simulink model "12_pulse_monopolar"  (R2021a)
settings: Solver=VariableStepAuto  StartTime=0.0  StopTime=2  MaxStep=1e-6  RelTol=1e-3
values from neighbouring files (symbols this model uses):
  alpha_i = 180 - gamma_min - mu    (= 160)    [link_params.m]
  alpha_r = 5    [link_params.m]
  V_AC_A = Vl_rms_A*ratio    (= 220000)    [link_params.m]
  V_AC_B = Vl_rms_B*ratio    (= 200000)    [link_params.m]
  Vl_rms_A = 22e3    (= 22000)    [link_params.m]
  Vl_rms_B = 20e3    (= 20000)    [link_params.m]
undefined symbols (not defined in the file or in its folder): D1, Delta, lagging, pulse
libraries: spsUniversalBridgeLib x4, spsSeriesRLCBranchLib x3, spsGroundLib x2, spsPLL3phLib x2, spsThreePhaseVIMeasurementLib x2, spsPulseGeneratorThyristor6PulseLib x2, spsTHDLib x2, spsThreePhaseTransformerThreeWindingsLib x2, spsThreePhaseSourceLib x2, spsVoltageMeasurementLib x2, spsCurrentMeasurementLib x1, spsMultimeterLib x1
settings Model: SimulationMode=accelerator  Creator=HossamAladdin  LastModifiedBy=HossamAladdin
settings DataIOCC: ReturnWorkspaceOutputs=off

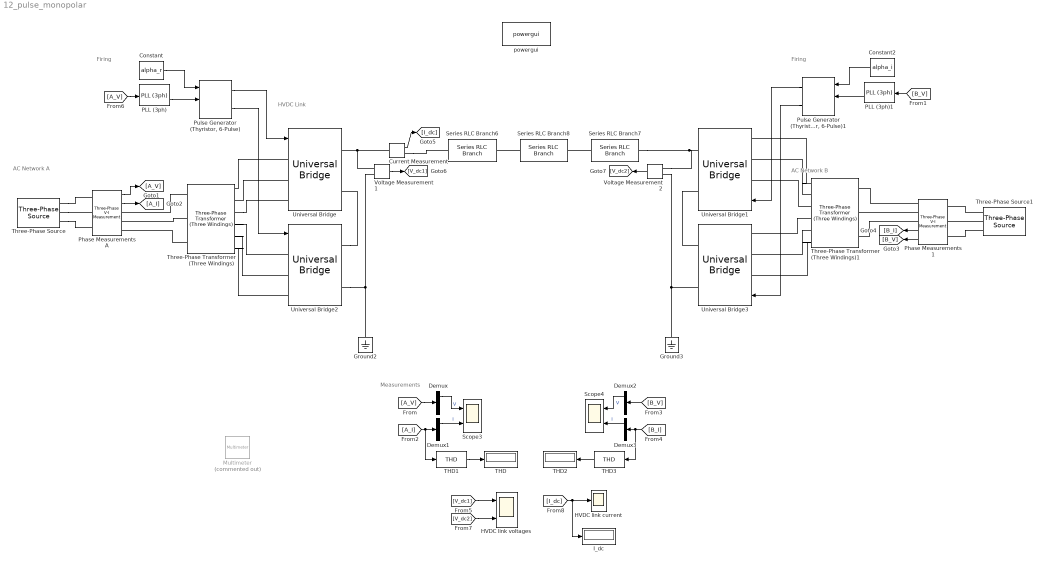
== system 12_pulse_monopolar ==
  note: Measurements
  note: HVDC Link
  note: AC Network A
  note: Firing
  note: AC Network B
  note: Firing
  Constant : Constant  Value=alpha_r
  Constant2 : Constant  Value=alpha_i
  Current Measurement : spsCurrentMeasurementLib/Current Measurement  PhasorSimulation=off  OutputType=Complex  PSBequivalent=0
  Demux{,1..3} (4 alike) : Demux  Outputs=3
  Ground2 : spsGroundLib/Ground  LConnTagsString=a
  Ground3 : spsGroundLib/Ground  LConnTagsString=a
  HVDC link current : Scope
  HVDC link voltages : Scope  NumInputPorts=2
  I_dc : Display
  Multimeter : spsMultimeterLib/Multimeter  Commented=on  PhasorSimulation=off  OutputType=Complex  sel=[1 7 11]  L=16  Gain=[1 1 1]  yselected={'Usw1: Universal Bridge1','Uab: Universal Bridge1','Isw1: Universal Bridge1'};  PSBOutputType=1  PSBequivalent=0  AxesSetting=[0,0.1,-100,100]  Display=1  SavedBlockNames=-11
  PLL (3ph) : spsPLL3phLib/PLL (3ph)  Fmin=50  Par_Init=[0, 50]  ParK=[180, 3200, 1]  TcD=1e-4  MaxRateChangeFreq=12  FilterCutOffFreq=25  Ts=0  AGC=on
  PLL (3ph)1 : spsPLL3phLib/PLL (3ph)  Fmin=60  Par_Init=[0, 60]  ParK=[180, 3200, 1]  TcD=1e-4  MaxRateChangeFreq=12  FilterCutOffFreq=25  Ts=0  AGC=on
  Phase Measurements A : spsThreePhaseVIMeasurementLib/Three-Phase V-I Measurement  VoltageMeasurement=phase-to-ground  SetLabelV=off  LabelV=Vabc  Vpu=off  VpuLL=off  CurrentMeasurement=yes  SetLabelI=off  LabelI=Iabc  Ipu=off  Pbase=100e6  Vbase=500e3  OutputType=Complex  PhasorSimulation=off  PSBequivalent=0
  Phase Measurements1 : spsThreePhaseVIMeasurementLib/Three-Phase V-I Measurement  VoltageMeasurement=phase-to-ground  SetLabelV=off  LabelV=Vabc  Vpu=off  VpuLL=off  CurrentMeasurement=yes  SetLabelI=off  LabelI=Iabc  Ipu=off  Pbase=100e6  Vbase=500e3  OutputType=Complex  PhasorSimulation=off  PSBequivalent=0
  "Pulse Generator (Thyristor, 6-Pulse)" : spsPulseGeneratorThyristor6PulseLib/Pulse Generator (Thyristor, 6-Pulse)  GenType=12-pulse  Delta=D1 (lagging)  pwidth=60  Double_Pulse=off  Ts=0
      settings: SourceProductBaseCode=PS
  "Pulse Generator (Thyristor, 6-Pulse)1" : spsPulseGeneratorThyristor6PulseLib/Pulse Generator (Thyristor, 6-Pulse)  GenType=12-pulse  Delta=D1 (lagging)  pwidth=60  Double_Pulse=off  Ts=0
      settings: SourceProductBaseCode=PS
  Scope3 : Scope  NumInputPorts=2
  Scope4 : Scope  NumInputPorts=2
  Series RLC Branch6 : spsSeriesRLCBranchLib/Series RLC Branch  LConnTagsString=__new0  RConnTagsString=__new0  BranchType=L  Resistance=1  Inductance=1.5  SetiL0=off  InitialCurrent=0  Capacitance=1e-6  Setx0=off  InitialVoltage=0  Measurements=None
  Series RLC Branch7 : spsSeriesRLCBranchLib/Series RLC Branch  LConnTagsString=__new0  RConnTagsString=__new0  BranchType=L  Resistance=1  Inductance=1.5  SetiL0=off  InitialCurrent=0  Capacitance=1e-6  Setx0=off  InitialVoltage=0  Measurements=None
  Series RLC Branch8 : spsSeriesRLCBranchLib/Series RLC Branch  LConnTagsString=__new0  RConnTagsString=__new0  BranchType=R  Resistance=10  Inductance=10e-3  SetiL0=off  InitialCurrent=0  Capacitance=1e-6  Setx0=off  InitialVoltage=0  Measurements=None
  THD : Display
  THD1 : spsTHDLib/THD  Freq=50  Ts=0
      settings: SourceProductBaseCode=PS
  THD2 : Display
  THD3 : spsTHDLib/THD  Freq=50  Ts=0
      settings: SourceProductBaseCode=PS
  Three-Phase Transformer (Three Windings) : spsThreePhaseTransformerThreeWindingsLib/Three-Phase Transformer (Three Windings)  Winding1Connection=Y  Winding2Connection=Y  Winding3Connection=Delta (D1)  CoreType=Three single-phase transformers  SetSaturation=off  Hysteresis=off  DataFile='hysteresis'  SetInitialFlux=off  Measurements=None  UNITS=SI  NominalPower=[ 1000e6 , 50 ]  Winding1=[Vl_rms_A 0 0]  Winding2=[V_AC_A/2 0 0]  Winding3=[V_AC_A/2 0.001 0]  Rm=inf  Lm=inf  L0=0.5  Saturation=[0 0;89.072 68.613;37113 86.91]  InitialFluxes=[-57.1777654238029 28.5888827119015 28.5888827119015]  BreakLoop=off  DiscreteSolver=Trapezoidal iterative  DataType=on  TransfoNumber=1
      settings: SourceProductBaseCode=PS
  Three-Phase Transformer (Three Windings)1 : spsThreePhaseTransformerThreeWindingsLib/Three-Phase Transformer (Three Windings)  Winding1Connection=Y  Winding2Connection=Delta (D1)  Winding3Connection=Y  CoreType=Three single-phase transformers  SetSaturation=off  Hysteresis=off  DataFile='hysteresis'  SetInitialFlux=off  Measurements=None  UNITS=SI  NominalPower=[ 1000e6 , 60 ]  Winding1=[Vl_rms_B 0 0]  Winding2=[V_AC_B/2 0.001 0]  Winding3=[V_AC_B/2 0 0]  Rm=inf  Lm=inf  L0=0.5  Saturation=[0 0;97.98 51.98;40825 65.841]  InitialFluxes=[0 64.9747334361397 64.9747334361397]  BreakLoop=off  DiscreteSolver=Trapezoidal iterative  DataType=on  TransfoNumber=1
      settings: SourceProductBaseCode=PS
  Three-Phase Source : spsThreePhaseSourceLib/Three-Phase Source  InternalConnection=Yg  VoltagePhases=off  Voltage=Vl_rms_A  PhaseAngle=0  Voltage_phases=[25e3 25e3 25e3]/sqrt(3)  PhaseAngles_phases=[0 -120 +120]  Frequency=50  NonIdealSource=off  SpecifyImpedance=off  Resistance=0.8929  Inductance=16.58e-3  ShortCircuitLevel=100e6  BaseVoltage=22e3  XRratio=7  BusType=swing  Pref=10e3  Qref=0  Prefabc=[10e3, 10e3, 10e3]  Qrefabc=[0, 0, 0]  Qmin=-inf  Qmax=inf
  Three-Phase Source1 : spsThreePhaseSourceLib/Three-Phase Source  InternalConnection=Yg  VoltagePhases=off  Voltage=Vl_rms_B  PhaseAngle=0  Voltage_phases=[25e3 25e3 25e3]/sqrt(3)  PhaseAngles_phases=[0 -120 +120]  Frequency=60  NonIdealSource=off  SpecifyImpedance=off  Resistance=0.8929  Inductance=16.58e-3  ShortCircuitLevel=100e6  BaseVoltage=20e3  XRratio=7  BusType=swing  Pref=10e3  Qref=0  Prefabc=[10e3, 10e3, 10e3]  Qrefabc=[0, 0, 0]  Qmin=-inf  Qmax=inf
  Universal Bridge : spsUniversalBridgeLib/Universal Bridge  Arms=3  SnubberResistance=1e5  SnubberCapacitance=inf  Device=Thyristors  Ron=Ron  Lon=0  ForwardVoltages="[  0  0  ]"  ForwardVoltage=0  GTOparameters=[ 10e-6 , 20e-6 ]  IGBTparameters=[ 1e-6 , 2e-6 ]  Measurements=None  Measurements_2=None  converterType=Rectifier
  Universal Bridge1 : spsUniversalBridgeLib/Universal Bridge  Arms=3  SnubberResistance=1e5  SnubberCapacitance=inf  Device=Thyristors  Ron=Ron  Lon=0  ForwardVoltages="[  0  0  ]"  ForwardVoltage=0  GTOparameters=[ 10e-6 , 20e-6 ]  IGBTparameters=[ 1e-6 , 2e-6 ]  Measurements=All voltages and currents  Measurements_2=None  converterType=Rectifier
  Universal Bridge2 : spsUniversalBridgeLib/Universal Bridge  Arms=3  SnubberResistance=1e5  SnubberCapacitance=inf  Device=Thyristors  Ron=Ron  Lon=0  ForwardVoltages="[  0  0  ]"  ForwardVoltage=0  GTOparameters=[ 10e-6 , 20e-6 ]  IGBTparameters=[ 1e-6 , 2e-6 ]  Measurements=None  Measurements_2=None  converterType=Rectifier
  Universal Bridge3 : spsUniversalBridgeLib/Universal Bridge  Arms=3  SnubberResistance=1e5  SnubberCapacitance=inf  Device=Thyristors  Ron=Ron  Lon=0  ForwardVoltages="[  0  0  ]"  ForwardVoltage=0  GTOparameters=[ 10e-6 , 20e-6 ]  IGBTparameters=[ 1e-6 , 2e-6 ]  Measurements=None  Measurements_2=None  converterType=Rectifier
  Voltage Measurement1 : spsVoltageMeasurementLib/Voltage Measurement  PhasorSimulation=off  OutputType=Complex  PSBequivalent=0
  Voltage Measurement2 : spsVoltageMeasurementLib/Voltage Measurement  PhasorSimulation=off  OutputType=Complex  PSBequivalent=0
  powergui : spspowerguiLib/powergui  Priority=1  SimulationMode=Discrete  SampleTime=1e-6  frequency=60  Iterations=50  frequencyindice=60  Pbase=100e6  ErrMax=1e-4  UnitsV=kV  UnitsW=MW  buscounter=0  FunctionMessages=off  echomessages=off  EnableUseOfTLC=off  CurrentSourceSwitches=off  DisableSnubberDevices=off  DisableRonSwitches=off  DisableVfSwitches=off  DisplayEquations=off  AutomaticDiscreteSolvers=off  SolverType=Tustin/Backward Euler (TBE)  Interpol=off  ExternalGateDelay=off  methode=off  Ts=100  x0status=blocks  SPID=on  SwTol=0  HookPort=off  NonlinearTolerance=1e-4  nMaxIteration=100  ContinueOnMaxIteration=off  RestoreLinks=warning  ResistiveCurrentMeasurement=off  Frange=[0:2:500]  Ylog=off  Xlog=on  ShowGrid=off  save=off  variable=ZData  structure=0  ZoomFFT=off  StartTime=0.0  cycles=1  DisplayStyle=1  fundamental=60  FreqAxis=off  MaxFrequency=1000  frequencyindicesteady=1  RmsSteady=1  display=off
  wires:
  Phase Measurements A/2 -> [A_I]
  Phase Measurements A/1 -> [A_V]
  [A_V] -> PLL (3ph)/1
  Constant/1 -> "Pulse Generator (Thyristor, 6-Pulse)"/1
  PLL (3ph)/2 -> "Pulse Generator (Thyristor, 6-Pulse)"/2
  "Pulse Generator (Thyristor, 6-Pulse)"/1 -> Universal Bridge/1
  Phase Measurements1/1 -> [B_V]
  Phase Measurements1/2 -> [B_I]
  [B_V] -> PLL (3ph)1/1
  PLL (3ph)1/2 -> "Pulse Generator (Thyristor, 6-Pulse)1"/2
  Constant2/1 -> "Pulse Generator (Thyristor, 6-Pulse)1"/1
  "Pulse Generator (Thyristor, 6-Pulse)1"/1 -> Universal Bridge1/1
  [A_V] -> Demux/1
  Demux/1 -> Scope3/1  "V"
  Demux1/1 -> Scope3/2  "I"
  [A_I] -> THD1/1, Demux1/1
  Demux2/1 -> Scope4/1  "V"
  [B_V] -> Demux2/1
  [B_I] -> THD3/1, Demux3/1
  Demux3/1 -> Scope4/2  "I"
  Current Measurement/1 -> [I_dc]
  Voltage Measurement1/1 -> [V_dc1]
  Voltage Measurement2/1 -> [V_dc2]
  [V_dc1] -> HVDC link voltages/1
  [V_dc2] -> HVDC link voltages/2
  [I_dc] -> HVDC link current/1, I_dc/1
  THD1/1 -> THD/1
  THD3/1 -> THD2/1
  "Pulse Generator (Thyristor, 6-Pulse)"/2 -> Universal Bridge2/1
  "Pulse Generator (Thyristor, 6-Pulse)1"/2 -> Universal Bridge3/1
  connections:
  Universal Bridge/LConn1 -- Three-Phase Transformer (Three Windings)/RConn1
  Universal Bridge/LConn2 -- Three-Phase Transformer (Three Windings)/RConn2
  Three-Phase Transformer (Three Windings)/RConn3 -- Universal Bridge/LConn3
  Three-Phase Transformer (Three Windings)/LConn3 -- Phase Measurements A/RConn3
  Three-Phase Transformer (Three Windings)/LConn2 -- Phase Measurements A/RConn2
  Three-Phase Transformer (Three Windings)/LConn1 -- Phase Measurements A/RConn1
  Series RLC Branch8/LConn1 -- Series RLC Branch6/RConn1
  Series RLC Branch7/LConn1 -- Series RLC Branch8/RConn1
  Current Measurement/LConn1 -- Voltage Measurement1/LConn1 -- Universal Bridge/RConn1
  Current Measurement/RConn1 -- Series RLC Branch6/LConn1
  Universal Bridge2/RConn1 -- Universal Bridge/RConn2
  Series RLC Branch7/RConn1 -- Voltage Measurement2/LConn2 -- Universal Bridge1/RConn2
  Universal Bridge3/RConn2 -- Universal Bridge1/RConn1
  Three-Phase Source1/RConn1 -- Phase Measurements1/LConn1
  Three-Phase Source1/RConn2 -- Phase Measurements1/LConn2
  Three-Phase Source1/RConn3 -- Phase Measurements1/LConn3
  Three-Phase Source/RConn1 -- Phase Measurements A/LConn1
  Three-Phase Source/RConn2 -- Phase Measurements A/LConn2
  Three-Phase Source/RConn3 -- Phase Measurements A/LConn3
  Universal Bridge2/RConn2 -- Voltage Measurement1/LConn2 -- Ground2/LConn1
  Universal Bridge3/RConn1 -- Voltage Measurement2/LConn1 -- Ground3/LConn1
  Three-Phase Transformer (Three Windings)/RConn6 -- Universal Bridge2/LConn3
  Three-Phase Transformer (Three Windings)/RConn5 -- Universal Bridge2/LConn2
  Three-Phase Transformer (Three Windings)/RConn4 -- Universal Bridge2/LConn1
  Phase Measurements1/RConn1 -- Three-Phase Transformer (Three Windings)1/LConn1
  Phase Measurements1/RConn2 -- Three-Phase Transformer (Three Windings)1/LConn2
  Phase Measurements1/RConn3 -- Three-Phase Transformer (Three Windings)1/LConn3
  Three-Phase Transformer (Three Windings)1/RConn1 -- Universal Bridge3/LConn1
  Three-Phase Transformer (Three Windings)1/RConn2 -- Universal Bridge3/LConn2
  Three-Phase Transformer (Three Windings)1/RConn3 -- Universal Bridge3/LConn3
  Three-Phase Transformer (Three Windings)1/RConn6 -- Universal Bridge1/LConn3
  Three-Phase Transformer (Three Windings)1/RConn5 -- Universal Bridge1/LConn2
  Three-Phase Transformer (Three Windings)1/RConn4 -- Universal Bridge1/LConn1
